simulink model "LgLf"  (R2022b)
settings: Solver=VariableStepAuto  StartTime=0.0  StopTime=10.0  RelTol=1e-3
settings Model: Creator=Milosh Yokich  LastModifiedBy=Milosh Yokich

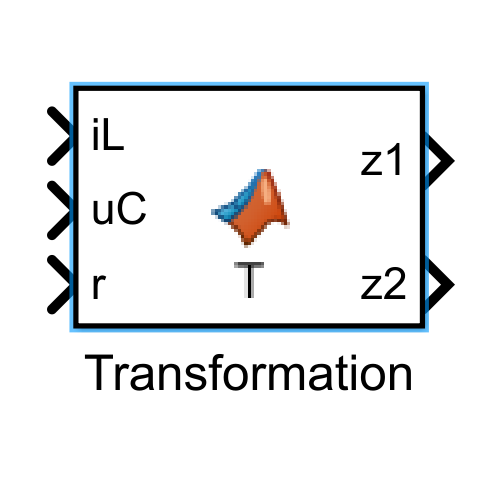
[thumbnail: Simulink's stored preview of the top-level diagram]
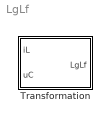
== system LgLf ==
  Transformation : MATLAB Function  TreatAsAtomicUnit=on

== matlab function LgLf/Transformation ==
  data: iL input; LgLf output; uC input
function LgLf = LgLf(iL, uC)
E = 12; %V
R = 52; %Omh
L = 0.01591; %H
C = 0.000470; %F 

LgLf = -E/L*(uC + E) + 1/(C*R)*iL*(E-2*uC);
